simulink model "test"  (R2024b)
settings: Solver=VariableStepAuto  StartTime=0.0  StopTime=inf  RelTol=1e-3
settings Model: Creator=kev  LastModifiedBy=kev

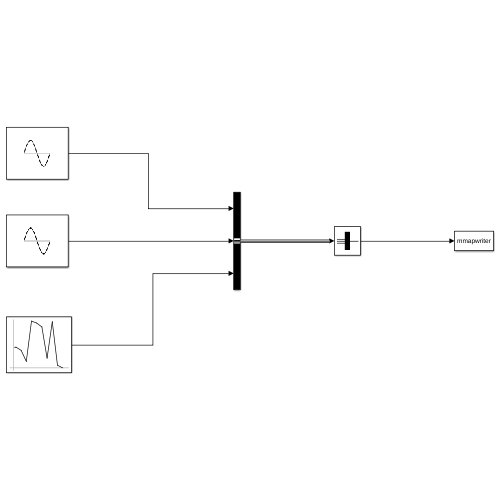
[thumbnail: Simulink's stored preview of the top-level diagram]
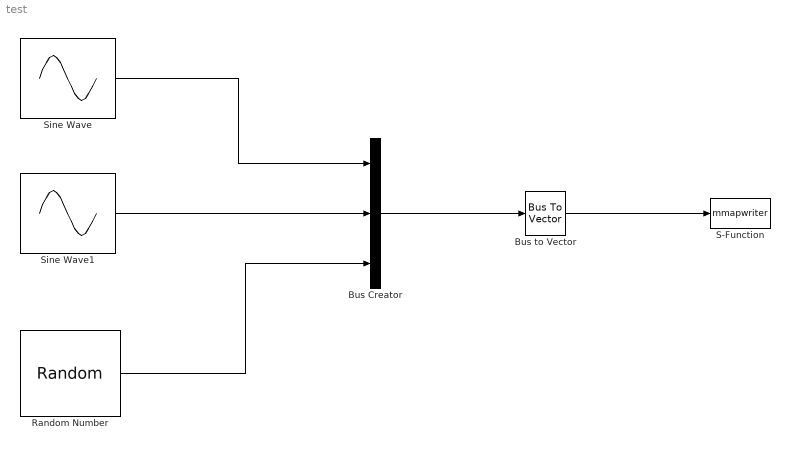
== system test ==
  Bus Creator : BusCreator  Inputs=3
  Bus to Vector : BusToVector
  Random Number : RandomNumber  SampleTime=0.1
  S-Function : S-Function  FunctionName=mmapwriter  Parameters='testing'  SFunctionDeploymentMode=off  EnableBusSupport=off
  Sine Wave : Sin  Amplitude=4  Frequency=2  SampleTime=0
  Sine Wave1 : Sin  SampleTime=0
  wires:
  Sine Wave/1 -> Bus Creator/1
  Sine Wave1/1 -> Bus Creator/2
  Random Number/1 -> Bus Creator/3
  Bus Creator/1 -> Bus to Vector/1
  Bus to Vector/1 -> S-Function/1
